simulink model "maglev_linear"  (R2024a)
settings: Solver=VariableStepAuto  StartTime=0.0  StopTime=tsim  RelTol=1e-3
values from neighbouring files (symbols this model uses):
  B = zeros(n,1)    [GetLinModFtxu.m]
  C = [0 1 0]    [sim_maglev.m]
  cden = den{:}    [sim_maglev.m]
  cnum = num{:}    [sim_maglev.m]
  ref = 0.025+0.001    (= 0.026)    [sim_maglev.m]
  xs = [is, ys, 0]    [sim_maglev.m]
undefined symbols (not defined in the file or in its folder): A
settings Model: Creator=Meenakshi Mahagaokar  LastModifiedBy=Meenakshi Mahagaokar
settings DataIOCC: SaveOutput=off  DSMLogging=off  SaveTime=off  ReturnWorkspaceOutputs=off

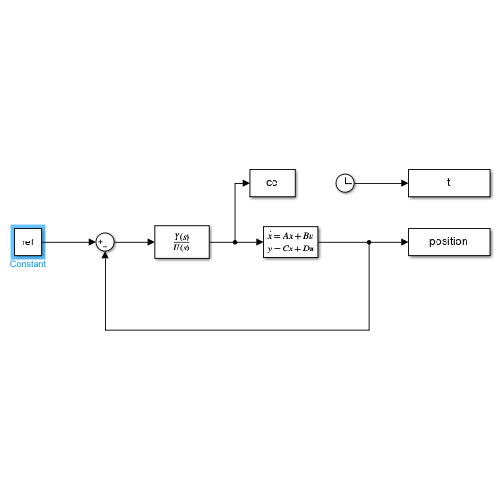
[thumbnail: Simulink's stored preview of the top-level diagram]
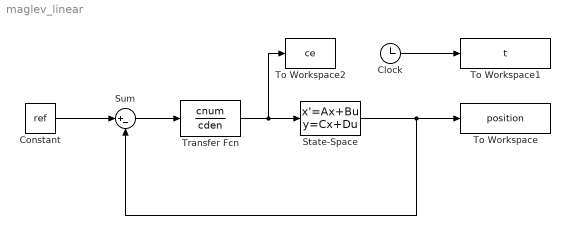
== system maglev_linear ==
  Clock : Clock
  Constant : Constant  Value=ref
  State-Space : StateSpace  A=A  B=B  C=C  D=0  InitialCondition=xs
  Sum : Sum  Inputs=|+-
  To Workspace : ToWorkspace  VariableName=position  SampleTime=-1
      settings: Save2DSignal=2-D array (concatenate along first dimension)
  To Workspace1 : ToWorkspace  VariableName=t  SampleTime=-1
      settings: Save2DSignal=2-D array (concatenate along first dimension)
  To Workspace2 : ToWorkspace  VariableName=ce  SampleTime=-1
      settings: Save2DSignal=2-D array (concatenate along first dimension)
  Transfer Fcn : TransferFcn  Numerator=cnum  Denominator=cden
  wires:
  Constant/1 -> Sum/1
  State-Space/1 -> Sum/2, To Workspace/1
  Clock/1 -> To Workspace1/1
  Sum/1 -> Transfer Fcn/1
  Transfer Fcn/1 -> To Workspace2/1, State-Space/1
